simulink model "MBD_week2_3"  (R2020b)
settings: Solver=VariableStepAuto  StartTime=0.0  StopTime=120  RelTol=1e-3
model workspace (MAT data in the model file):
  B = Simulink.Parameter
  B.Value = 50
  B.DataType = 'auto'
  B.Dimensions = [1 1]
  Kd = Simulink.Parameter
  Kd.Value = 484.0516
  Kd.DataType = 'auto'
  Kd.Dimensions = [1 1]
  Ki = Simulink.Parameter
  Ki.Value = 83.0917
  Ki.DataType = 'auto'
  Ki.Dimensions = [1 1]
  Kp = Simulink.Parameter
  Kp.Value = 495.0505
  Kp.DataType = 'auto'
  Kp.Dimensions = [1 1]
  M = Simulink.Parameter
  M.Value = 1000
  M.DataType = 'auto'
  M.Dimensions = [1 1]
settings Model: Creator=varunraj  LastModifiedBy=varunraj

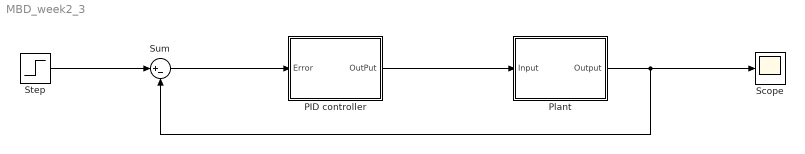
== system MBD_week2_3 ==
  PID controller : Subsystem  TreatAsAtomicUnit=on
  Plant : Subsystem
  Scope : Scope
  Step : Step  After=10  SampleTime=0
  Sum : Sum  Inputs=|+-
  wires:
  Step/1 -> Sum/1
  Sum/1 -> PID controller/1(Error)
  PID controller/1(OutPut) -> Plant/1(Input)
  Plant/1(Output) -> Scope/1, Sum/2

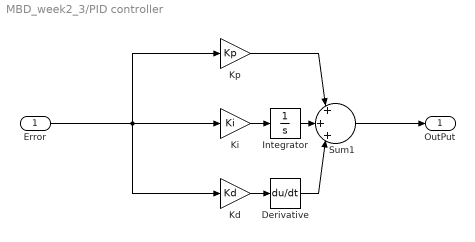
== system MBD_week2_3/PID controller ==
  Error : Inport  OutDataTypeStr=double  PortDimensions=1  SampleTime=0
  Derivative : Derivative
  Integrator : Integrator
  Kd : Gain  Gain=Kd
  Ki : Gain  Gain=Ki
  Kp : Gain  Gain=Kp
  Sum1 : Sum  Inputs=|+|+|+|
  OutPut : Outport  OutDataTypeStr=double  PortDimensions=1  SampleTime=0
  wires:
  Ki/1 -> Integrator/1
  Kd/1 -> Derivative/1
  Kp/1 -> Sum1/1
  Sum1/1 -> OutPut/1
  Error/1 -> Kd/1, Kp/1, Ki/1
  Derivative/1 -> Sum1/3
  Integrator/1 -> Sum1/2

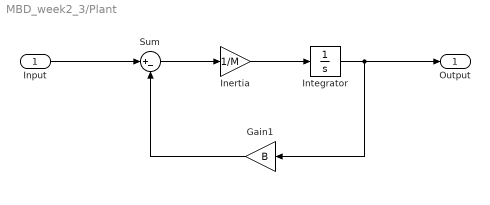
== system MBD_week2_3/Plant ==
  Input : Inport
  Gain1 : Gain  Gain=B
  Inertia : Gain  Gain=1/M
  Integrator : Integrator
  Sum : Sum  Inputs=|+-
  Output : Outport
  wires:
  Sum/1 -> Inertia/1
  Integrator/1 -> Output/1, Gain1/1
  Gain1/1 -> Sum/2
  Inertia/1 -> Integrator/1
  Input/1 -> Sum/1
